simulink model "activecellbalancingusingflybackconverters"  (R2023a)
settings: Solver=VariableStepAuto  StartTime=0.0  StopTime=700  RelTol=1e-3
libraries: spsVoltageMeasurementLib x4, spsDiodeLib x2, spsSeriesRLCBranchLib x2, spsGroundLib x1, spsLinearTransformerLib x1, spsMosfetLib x1, spspowerguiLib x1
settings Model: Creator=animesh184  LastModifiedBy=animesh184

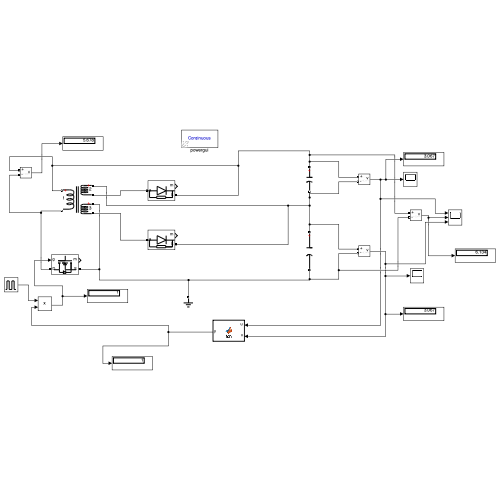
[thumbnail: Simulink's stored preview of the top-level diagram]
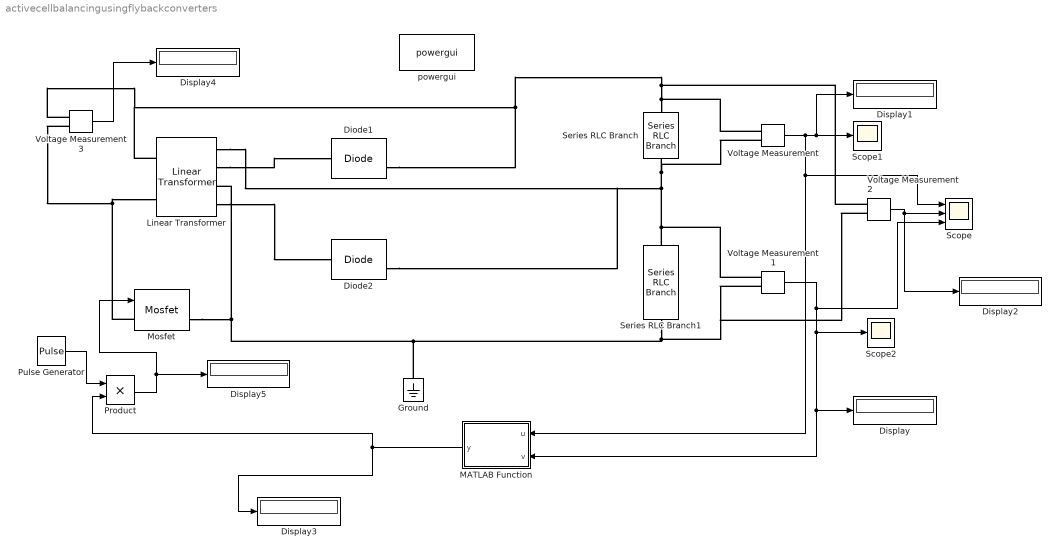
== system activecellbalancingusingflybackconverters ==
  Diode1 : spsDiodeLib/Diode  Ron=0.001  Lon=0  Vf=0.8  IC=0  UseSnubber=0  Rs=500  Cs=250e-9  Measurements=on
  Diode2 : spsDiodeLib/Diode  Ron=0.001  Lon=0  Vf=0.8  IC=0  UseSnubber=0  Rs=500  Cs=250e-9  Measurements=on
  Display{,1..5} (6 alike) : Display
  Ground : spsGroundLib/Ground  LConnTagsString=a
  Linear Transformer : spsLinearTransformerLib/Linear Transformer  UNITS=SI  NominalPower=[ 100 55000 ]  winding1=[10 0.02 45e-6]  winding2=[5 0.02 288e-6]  ThreeWindings=on  winding3=[5 0.02 288e-6]  RmLm=[1.0805e+06 2866]  Measurements=None  DataType=on
  MATLAB Function : MATLAB Function  TreatAsAtomicUnit=on
  Mosfet : spsMosfetLib/Mosfet  Ron=1.5  Lon=0  Rd=2  Vfd=0  IC=0  Rs=1500  Cs=288e-7  Measurements=on
  Product : Product
  Pulse Generator : DiscretePulseGenerator  PulseType=Time based  Period=10  PulseWidth=50
  Scope : Scope  NumInputPorts=3
  Scope1 : Scope
  Scope2 : Scope
  Series RLC Branch : spsSeriesRLCBranchLib/Series RLC Branch  LConnTagsString=__new0  RConnTagsString=__new0  BranchType=C  Resistance=1  Inductance=1e-3  SetiL0=off  InitialCurrent=0  Capacitance=5  Setx0=on  InitialVoltage=3  Measurements=None
  Series RLC Branch1 : spsSeriesRLCBranchLib/Series RLC Branch  LConnTagsString=__new0  RConnTagsString=__new0  BranchType=C  Resistance=1  Inductance=1e-3  SetiL0=off  InitialCurrent=0  Capacitance=5  Setx0=on  InitialVoltage=3.3  Measurements=None
  Voltage Measurement{,1..3} (4 alike) : spsVoltageMeasurementLib/Voltage Measurement  PhasorSimulation=off  OutputType=Complex  PSBequivalent=0
  powergui : spspowerguiLib/powergui  Priority=1  SimulationMode=Continuous  SampleTime=50e-6  frequency=60  Iterations=50  frequencyindice=0  Pbase=100e6  ErrMax=1e-4  UnitsV=kV  UnitsW=MW  buscounter=0  FunctionMessages=off  echomessages=off  EnableUseOfTLC=off  CurrentSourceSwitches=off  DisableSnubberDevices=off  DisableRonSwitches=off  DisableVfSwitches=off  DisplayEquations=off  AutomaticDiscreteSolvers=off  SolverType=Tustin/Backward Euler (TBE)  Interpol=off  ExternalGateDelay=off  methode=off  Ts=100  x0status=blocks  SPID=on  SwTol=0  HookPort=off  NonlinearTolerance=1e-4  nMaxIteration=100  ContinueOnMaxIteration=off  RestoreLinks=warning  ResistiveCurrentMeasurement=off  Frange=[0:2:500]  Ylog=off  Xlog=on  ShowGrid=off  save=off  variable=ZData  structure=0  ZoomFFT=off  StartTime=0.0  cycles=1  DisplayStyle=1  fundamental=60  FreqAxis=off  MaxFrequency=1000  frequencyindicesteady=1  RmsSteady=1  display=off
  wires:
  Pulse Generator/1 -> Product/1
  Product/1 -> Display5/1, Mosfet/1
  MATLAB Function/1(y) -> Product/2, Display3/1
  Voltage Measurement2/1 -> Display2/1, Scope/2
  Voltage Measurement/1 -> Scope/1, MATLAB Function/1(u), Display1/1, Scope1/1
  Voltage Measurement1/1 -> Scope/3, Scope2/1, MATLAB Function/2(v), Display/1
  Voltage Measurement3/1 -> Display4/1
  connections:
  Series RLC Branch1/LConn1 -- Voltage Measurement1/LConn1 -- Diode2/RConn1 -- Linear Transformer/RConn1 -- Voltage Measurement/LConn2 -- Series RLC Branch/RConn1
  Linear Transformer/RConn2 -- Diode1/LConn1
  Diode1/RConn1 -- Linear Transformer/LConn1 -- Voltage Measurement3/LConn1 -- Voltage Measurement2/LConn1 -- Voltage Measurement/LConn1 -- Series RLC Branch/LConn1
  Linear Transformer/RConn4 -- Diode2/LConn1
  Mosfet/LConn1 -- Voltage Measurement3/LConn2 -- Linear Transformer/LConn2
  Series RLC Branch1/RConn1 -- Voltage Measurement2/LConn2 -- Voltage Measurement1/LConn2 -- Ground/LConn1 -- Mosfet/RConn1 -- Linear Transformer/RConn3

== matlab function activecellbalancingusingflybackconverters/MATLAB Function ==
  data: u input; y output; v input
function y  = fcn(u,v)

if (u <= v && v <= u)
    y=0;
else
    y=1;
end
